simulink model "SimscapeFoundation_singleDiodeModel_solarCell"  (R2017b)
settings: Solver=FixedStepDiscrete  StartTime=0.0  StopTime=3.5  FixedStep=0.0001  MaxStep=1e-4  RelTol=1e-3
StopFcn:
  | run('plot_IV_curve')
undefined symbols (not defined in the file): physconst
libraries: fl_lib x5, nesl_utility x5, simulink x2
settings Model: Creator=Adrian  LastModifiedBy=Adrian

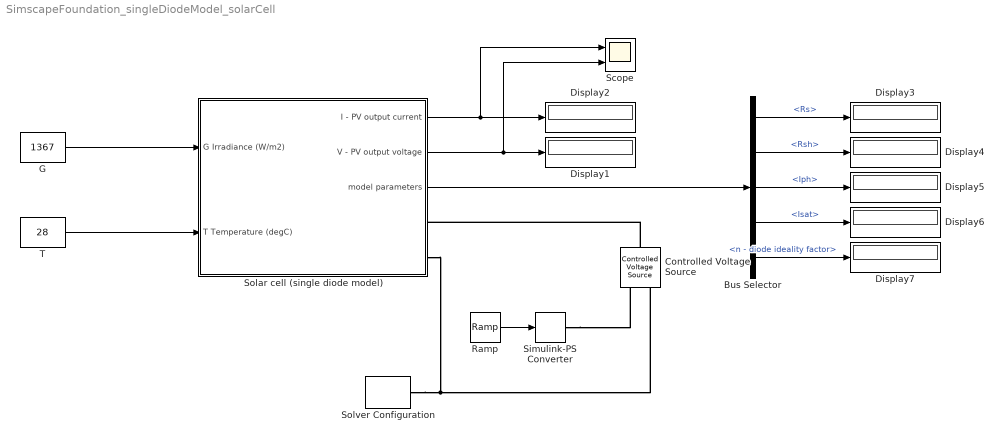
== system SimscapeFoundation_singleDiodeModel_solarCell ==
  Bus Selector : BusSelector  OutputSignals=Rs,Rsh,Iph,Isat,n - diode ideality factor
  Controlled Voltage Source : fl_lib/Electrical/Electrical Sources/Controlled Voltage Source
  Display{1..7} (7 alike) : Display
  G : Constant  Value=1367
  Ramp : simulink/Sources/Ramp  slope=1  start=0  X0=0
  Scope : Scope  NumInputPorts=2
  Simulink-PS Converter : nesl_utility/Simulink-PS Converter  PhysicalDomain=network_engine_domain  SubClassName=ps_input  LeftPortType=input  RightPortType=output  PseudoPeriodic=off  Frequencies=[]  NoiseDistribution=none  NoiseParameters=[]  Unit=1  AffineConversion=off  FilteringAndDerivatives=provide  SimscapeFilterOrder=1  InputFilterTimeConstant=0.001  UdotUserProvided=0
  Solar cell (single diode model) : Subsystem  mask(Solar cell model){T_ref=28, G_ref=1367, Voc_ref=2512, Isc_ref=501.3, Vmpp_ref=2244, Impp_ref=485.1, DVoc=-6.7, DVmpp=-7.2, DIsc=0.38, DImpp=0.28}
      mask prompts: T_ref "Temperature (degC), T_ref ="; G_ref "Irradiation (W/m2), G_ref ="; Voc_ref "Open circuit voltage (mV), Voc ="; Isc_ref "Short circuit current (mA), Isc ="; Vmpp_ref "Voltage @ mpp (mV), Vmpp ="; Impp_ref "Current @ mpp (mA), Impp ="; DVoc "Delta Voc / Delta T (mV/degC), DVoc ="; DVmpp "Delta Vmpp / Delta T (mV/degC), DVmpp ="; DIsc "Delta Isc / Delta T (mA/degC), DIsc ="; DImpp "Delta Impp / Delta T (mA/degC), DImpp ="
      mask help:
      | - "single diode + inner losses" solar cell model
      | - setup: current source, parallel diode, shunt and series resistor
      | - calculating the solar cell model's 5 parameters (Iph, Isat, n, Rsh, Rs, where n is already given) on every time step
      | - using those 5 parameters to control a parametrized current source
      | - input: irradiance, temperature
      | - model parameters get determined by using Voc, Isc, V and I @ mpp and the corresponding temperature dependencies of the given (modeled) solar cell
      mask TypeOptions T_ref: calculate 5 parameters of single diode solar cell model/T_ref
      mask TypeOptions G_ref: calculate 5 parameters of single diode solar cell model/G_ref
      mask TypeOptions Voc_ref: calculate 5 parameters of single diode solar cell model/Voc_ref
      mask TypeOptions Isc_ref: calculate 5 parameters of single diode solar cell model/Isc_ref
      mask TypeOptions Vmpp_ref: calculate 5 parameters of single diode solar cell model/Vmpp_ref
      mask TypeOptions Impp_ref: calculate 5 parameters of single diode solar cell model/Impp_ref
      mask TypeOptions DVoc: calculate 5 parameters of single diode solar cell model/DVoc
      mask TypeOptions DVmpp: calculate 5 parameters of single diode solar cell model/DVmpp
      mask TypeOptions DIsc: calculate 5 parameters of single diode solar cell model/DIsc
      mask TypeOptions DImpp: calculate 5 parameters of single diode solar cell model/DImpp
      mask DialogControl ParameterGroupVar Prompt: Conditions of reference measurement
      mask DialogControl Container3 Prompt: Characteristics (reference measurement @ T_ref, G_ref)
      mask DialogControl Container4 Prompt: Temperature dependencies
  Solver Configuration : nesl_utility/Solver Configuration  PhysicalDomain=network_engine_domain  SubClassName=solver  LeftPortType=input  RightPortType=generic  Accelerate=off  Tones=[]  Harmonics=[]  SimulateNoise=off  Profile=off  UseLocalSampling=off  EnableSwitchedLinearOptims=on  FrequencyDomain=off  UseCCode=off  RelTol=0.001  AbsTol=1e-06  MinStep=1e-09  ToWorkspace=off  RevertToSquareIcSolve=off  NumHomotopyIterations=100  PhasorMode=off  PhasorModeNumHarmonics=1  DoDC=off  ResidualTolerance=1e-09  UseLocalSolver=on  LocalSolverChoice=NE_BACKWARD_EULER_ADVANCER  LocalSolverSampleTime=0.001  DoFixedCost=on  MaxNonlinIter=3  MaxModeIter=2  LinearAlgebra=Sparse  DelaysMemoryBudget=1024  AutomaticFiltering=on  FilteringTimeConstant=0.001
  T : Constant  Value=28
  wires:
  G/1 -> Solar cell (single diode model)/1(G Irradiance (W/m2))
  T/1 -> Solar cell (single diode model)/2(T Temperature (degC))
  Solar cell (single diode model)/2(V - PV output voltage) -> Scope/2, Display1/1
  Solar cell (single diode model)/1(I - PV output current) -> Scope/1, Display2/1
  Ramp/1 -> Simulink-PS Converter/1
  Solar cell (single diode model)/3(model parameters) -> Bus Selector/1
  Bus Selector/1 -> Display3/1  "<Rs>"
  Bus Selector/2 -> Display4/1  "<Rsh>"
  Bus Selector/3 -> Display5/1  "<Iph>"
  Bus Selector/4 -> Display6/1  "<Isat>"
  Bus Selector/5 -> Display7/1  "<n - diode ideality factor>"
  connections:
  Controlled Voltage Source/LConn1 -- Solar cell (single diode model)/RConn1
  Solar cell (single diode model)/RConn2 -- Solver Configuration/RConn1 -- Controlled Voltage Source/RConn2
  Simulink-PS Converter/RConn1 -- Controlled Voltage Source/RConn1

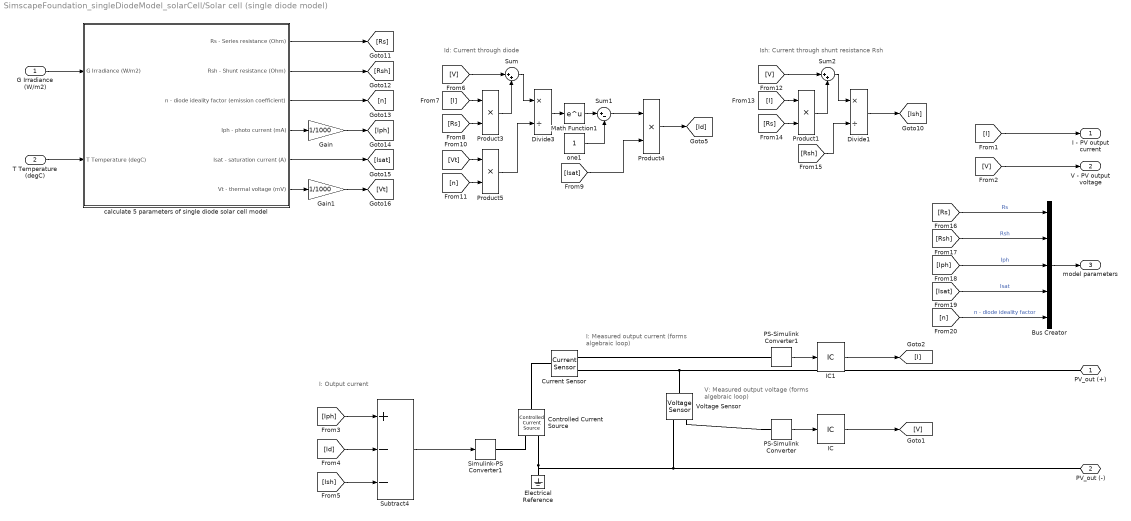
== system SimscapeFoundation_singleDiodeModel_solarCell/Solar cell (single diode model) ==
  note: Id: Current through diode
  note: Ish: Current through shunt resistance Rsh
  note: I: Output current
  note: I: Measured output current
      | (forms algebraic loop)
  note: V: Measured output voltage
      | (forms algebraic loop)
  G Irradiance (W/m2) : Inport
  T Temperature (degC) : Inport  Port=2
  Bus Creator : BusCreator  Inputs=5
  Controlled Current Source : fl_lib/Electrical/Electrical Sources/Controlled Current Source
  Current Sensor : fl_lib/Electrical/Electrical Sensors/Current Sensor
  Divide1 : Product  Inputs=*/
  Divide3 : Product  Inputs=*/
  Electrical Reference : fl_lib/Electrical/Electrical Elements/Electrical Reference
  Gain : Gain  Gain=1/1000
  Gain1 : Gain  Gain=1/1000
  IC : InitialCondition  Value=2.5
  IC1 : InitialCondition  Value=0.02
  Math Function1 : Math  SaturateOnIntegerOverflow=on
  PS-Simulink Converter : nesl_utility/PS-Simulink Converter  PhysicalDomain=network_engine_domain  SubClassName=ps_output  LeftPortType=input  RightPortType=output  PseudoPeriodic=off  Frequencies=[]  Unit=1  AffineConversion=off
  PS-Simulink Converter1 : nesl_utility/PS-Simulink Converter  PhysicalDomain=network_engine_domain  SubClassName=ps_output  LeftPortType=input  RightPortType=output  PseudoPeriodic=off  Frequencies=[]  Unit=1  AffineConversion=off
  Product{1,3..5} (4 alike) : Product
  Simulink-PS Converter1 : nesl_utility/Simulink-PS Converter  PhysicalDomain=network_engine_domain  SubClassName=ps_input  LeftPortType=input  RightPortType=output  PseudoPeriodic=off  Frequencies=[]  NoiseDistribution=none  NoiseParameters=[]  Unit=1  AffineConversion=off  FilteringAndDerivatives=provide  SimscapeFilterOrder=1  InputFilterTimeConstant=0.001  UdotUserProvided=0
  Subtract4 : Sum  Inputs=+--
  Sum : Sum  Inputs=|++
  Sum1 : Sum  Inputs=|+-
  Sum2 : Sum  Inputs=|++
  Voltage Sensor : fl_lib/Electrical/Electrical Sensors/Voltage Sensor
  calculate 5 parameters of single diode solar cell model : Subsystem  mask(Parameter identifier of "single diode" solar cell model){n=1.5, T_ref=T_ref, G_ref=G_ref, Voc_ref=Voc_ref, Isc_ref=Isc_ref, Vmpp_ref=Vmpp_ref, Impp_ref=Impp_ref, DVoc=DVoc, DVmpp=DVmpp, DIsc=DIsc, DImpp=DImpp}
      mask prompts: n "Diode ideality factor (emission coefficient)"; T_ref "Temperature (degC), T_ref ="; G_ref "Irradiation (W/m2), G_ref ="; Voc_ref "Open circuit voltage (mV), Voc ="; Isc_ref "Short circuit current (mA), Isc ="; Vmpp_ref "Voltage @ mpp (mV), Vmpp ="; Impp_ref "Current @ mpp (mA), Impp ="; DVoc "Delta Voc / Delta T (mV/degC), DVoc ="; DVmpp "Delta Vmpp / Delta T (mV/degC), DVmpp ="; DIsc "Delta Isc / Delta T (mA/degC), DIsc ="; DImpp "Delta Impp / Delta T (mA/degC), DImpp ="
      mask help:
      | - solar cell model, type: single diode + innert losses
      | - using a current source, parallel diode, shunt and series resistor
      | - output: 5 parameters (Iph, Isat, n, Rsh, Rs)
      | - input: irradiance, temperature
      | - model parameters get determined by using Voc, Isc, V and I @ mpp and the corresponding temperature dependencies
      mask DialogControl Container5 Prompt: Tunable model parameters
      mask DialogControl ParameterGroupVar Prompt: Conditions of reference measurement
      mask DialogControl Container8 Prompt: Characteristics (reference measurement @ T_ref, G_ref)
      mask DialogControl Container9 Prompt: Temperature dependencies
  one1 : Constant
  PV_out (+) : PMIOPort  Port=1  Side=Right
  PV_out (-) : PMIOPort  Port=2  Side=Right
  I - PV output current : Outport
  V - PV output voltage : Outport  Port=2
  model parameters : Outport  Port=3
  wires:
  Gain/1 -> [Iph]
  [I] -> Product1/1
  Product1/1 -> Sum2/2
  [V] -> Sum2/1
  [Id] -> Subtract4/2
  Divide3/1 -> Math Function1/1
  one1/1 -> Sum1/2
  Sum/1 -> Divide3/1
  [V] -> Sum/1
  [Ish] -> Subtract4/3
  Sum1/1 -> Product4/1
  Subtract4/1 -> Simulink-PS Converter1/1
  [Rs] -> Product1/2
  Product3/1 -> Sum/2
  PS-Simulink Converter/1 -> IC/1
  PS-Simulink Converter1/1 -> IC1/1
  Math Function1/1 -> Sum1/1
  [Isat] -> Product4/2
  [Rsh] -> Divide1/2
  Product4/1 -> [Id]
  [Vt] -> Product5/1
  [n] -> Product5/2
  [Iph] -> Subtract4/1
  [I] -> Product3/1
  Product5/1 -> Divide3/2
  IC/1 -> [V]
  IC1/1 -> [I]
  calculate 5 parameters of single diode solar cell model/6(Vt - thermal voltage (mV)) -> Gain1/1
  calculate 5 parameters of single diode solar cell model/4(Iph - photo current (mA)) -> Gain/1
  calculate 5 parameters of single diode solar cell model/1(Rs - Series resistance (Ohm)) -> [Rs]
  calculate 5 parameters of single diode solar cell model/5(Isat - saturation current (A)) -> [Isat]
  Sum2/1 -> Divide1/1
  Divide1/1 -> [Ish]
  calculate 5 parameters of single diode solar cell model/2(Rsh - Shunt resistance (Ohm)) -> [Rsh]
  T Temperature (degC)/1 -> calculate 5 parameters of single diode solar cell model/2(T Temperature (degC))
  Gain1/1 -> [Vt]
  [Rs] -> Product3/2
  G Irradiance (W/m2)/1 -> calculate 5 parameters of single diode solar cell model/1(G Irradiance (W/m2))
  calculate 5 parameters of single diode solar cell model/3(n - diode ideality factor (emission coefficient)) -> [n]
  [I] -> I - PV output current/1
  [V] -> V - PV output voltage/1
  [Rs] -> Bus Creator/1  "Rs"
  [Rsh] -> Bus Creator/2  "Rsh"
  [Iph] -> Bus Creator/3  "Iph"
  [Isat] -> Bus Creator/4  "Isat"
  Bus Creator/1 -> model parameters/1
  [n] -> Bus Creator/5  "n - diode ideality factor"
  connections:
  Controlled Current Source/LConn1 -- Current Sensor/LConn1
  Simulink-PS Converter1/RConn1 -- Controlled Current Source/RConn1
  Voltage Sensor/RConn2 -- PV_out (-)/RConn1 -- Electrical Reference/LConn1 -- Controlled Current Source/RConn2
  PS-Simulink Converter/LConn1 -- Voltage Sensor/RConn1
  Current Sensor/RConn2 -- Voltage Sensor/LConn1 -- PV_out (+)/RConn1
  Current Sensor/RConn1 -- PS-Simulink Converter1/LConn1

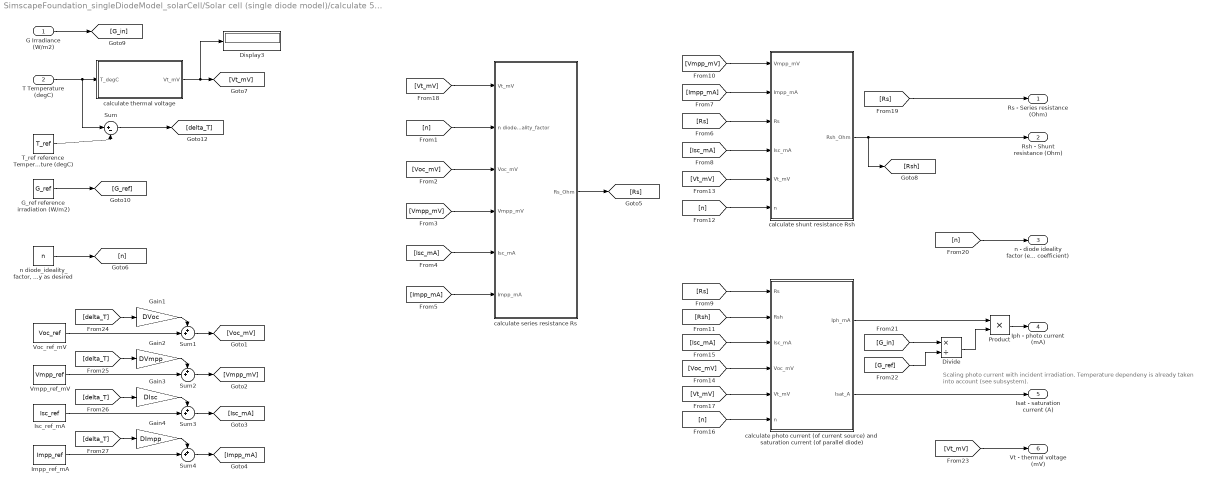
== system SimscapeFoundation_singleDiodeModel_solarCell/Solar cell (single diode model)/calculate 5 parameters of single diode solar cell model ==
  note: Scaling photo current with incident irradiation.
      | Temperature dependeny is already taken into account (see subsystem).
  G Irradiance (W/m2) : Inport
  T Temperature (degC) : Inport  Port=2
  Display3 : Display
  Divide : Product  Inputs=*/
  G_ref reference irradiation (W/m2) : Constant  Value=G_ref
  Gain1 : Gain  Gain=DVoc
  Gain2 : Gain  Gain=DVmpp
  Gain3 : Gain  Gain=DIsc
  Gain4 : Gain  Gain=DImpp
  Impp_ref_mA : Constant  Value=Impp_ref
  Isc_ref_mA : Constant  Value=Isc_ref
  Product : Product
  Sum : Sum  Inputs=|+-
  Sum{1..4} (4 alike) : Sum  Inputs=++|
  T_ref reference Temperature (degC) : Constant  Value=T_ref
  Vmpp_ref_mV : Constant  Value=Vmpp_ref
  Voc_ref_mV : Constant  Value=Voc_ref
  calculate photo current (of current source) and saturation current (of parallel diode) : Subsystem
  calculate series resistance Rs : Subsystem
  calculate shunt resistance Rsh : Subsystem
  calculate thermal voltage : Subsystem
  "n diode_ideality_factor, normally 1...2 specify as desired " : Constant  Value=n
  Rs - Series resistance (Ohm) : Outport
  Rsh - Shunt resistance (Ohm) : Outport  Port=2
  n - diode ideality factor (emission coefficient) : Outport  Port=3
  Iph - photo current (mA) : Outport  Port=4
  Isat - saturation current (A) : Outport  Port=5
  Vt - thermal voltage (mV) : Outport  Port=6
  wires:
  [Vt_mV] -> calculate series resistance Rs/1(Vt_mV)
  [Impp_mA] -> calculate series resistance Rs/6(Impp_mA)
  [Vmpp_mV] -> calculate series resistance Rs/4(Vmpp_mV)
  [Isc_mA] -> calculate series resistance Rs/5(Isc_mA)
  [Voc_mV] -> calculate series resistance Rs/3(Voc_mV)
  calculate thermal voltage/1(Vt_mV) -> Display3/1, [Vt_mV]
  [n] -> calculate series resistance Rs/2(n diode_ideality_factor)
  calculate series resistance Rs/1(Rs_Ohm) -> [Rs]
  "n diode_ideality_factor, normally 1...2 specify as desired "/1 -> [n]
  [n] -> calculate shunt resistance Rsh/6(n)
  [Rs] -> calculate photo current (of current source) and saturation current (of parallel diode)/1(Rs)
  calculate photo current (of current source) and saturation current (of parallel diode)/2(Isat_A) -> Isat - saturation current (A)/1
  [Voc_mV] -> calculate photo current (of current source) and saturation current (of parallel diode)/4(Voc_mV)
  [Impp_mA] -> calculate shunt resistance Rsh/2(Impp_mA)
  [Vt_mV] -> calculate shunt resistance Rsh/5(Vt_mV)
  [Vt_mV] -> calculate photo current (of current source) and saturation current (of parallel diode)/5(Vt_mV)
  [Rs] -> calculate shunt resistance Rsh/3(Rs)
  [Isc_mA] -> calculate shunt resistance Rsh/4(Isc_mA)
  [Vmpp_mV] -> calculate shunt resistance Rsh/1(Vmpp_mV)
  [Isc_mA] -> calculate photo current (of current source) and saturation current (of parallel diode)/3(Isc_mA)
  [n] -> calculate photo current (of current source) and saturation current (of parallel diode)/6(n)
  [Rsh] -> calculate photo current (of current source) and saturation current (of parallel diode)/2(Rsh)
  calculate shunt resistance Rsh/1(Rsh_Ohm) -> Rsh - Shunt resistance (Ohm)/1, [Rsh]
  calculate photo current (of current source) and saturation current (of parallel diode)/1(Iph_mA) -> Product/1
  T Temperature (degC)/1 -> Sum/1, calculate thermal voltage/1(T_degC)
  [Rs] -> Rs - Series resistance (Ohm)/1
  G Irradiance (W/m2)/1 -> [G_in]
  [G_in] -> Divide/1
  [n] -> n - diode ideality factor (emission coefficient)/1
  Product/1 -> Iph - photo current (mA)/1
  G_ref reference irradiation (W/m2)/1 -> [G_ref]
  Divide/1 -> Product/2
  [G_ref] -> Divide/2
  [Vt_mV] -> Vt - thermal voltage (mV)/1
  T_ref reference Temperature (degC)/1 -> Sum/2
  Sum/1 -> [delta_T]
  [delta_T] -> Gain1/1
  Voc_ref_mV/1 -> Sum1/2
  Sum1/1 -> [Voc_mV]
  Gain1/1 -> Sum1/1
  Gain2/1 -> Sum2/1
  Sum2/1 -> [Vmpp_mV]
  Vmpp_ref_mV/1 -> Sum2/2
  [delta_T] -> Gain2/1
  [delta_T] -> Gain4/1
  Impp_ref_mA/1 -> Sum4/2
  Sum4/1 -> [Impp_mA]
  Gain4/1 -> Sum4/1
  Gain3/1 -> Sum3/1
  Sum3/1 -> [Isc_mA]
  Isc_ref_mA/1 -> Sum3/2
  [delta_T] -> Gain3/1

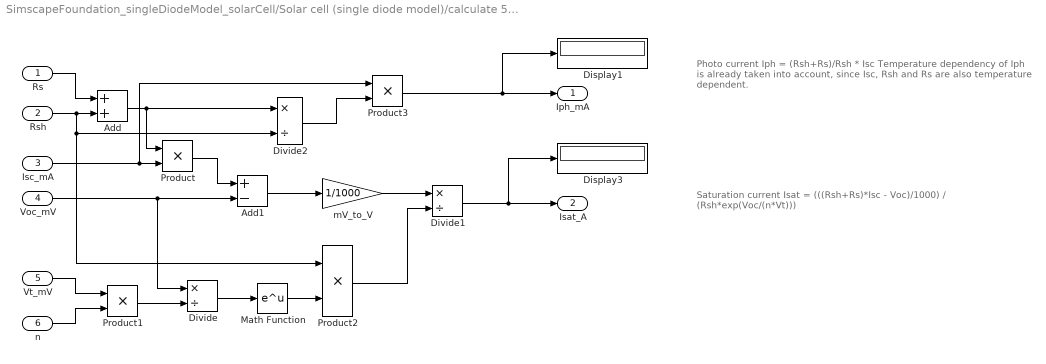
== system SimscapeFoundation_singleDiodeModel_solarCell/Solar cell (single diode model)/calculate 5 parameters of single diode solar cell model/calculate photo current (of current source) and saturation current (of parallel diode) ==
  note: Saturation current
      | Isat = (((Rsh+Rs)*Isc - Voc)/1000) / (Rsh*exp(Voc/(n*Vt)))
  note: Photo current
      | Iph = (Rsh+Rs)/Rsh * Isc
      |
      | Temperature dependency of Iph is already taken into account,
      | since Isc, Rsh and Rs are also temperature dependent.
  Rs : Inport
  Rsh : Inport  Port=2
  Isc_mA : Inport  Port=3
  Voc_mV : Inport  Port=4
  Vt_mV : Inport  Port=5
  n : Inport  Port=6
  Add : Sum
  Add1 : Sum  Inputs=+-
  Display1 : Display
  Display3 : Display
  Divide : Product  Inputs=*/
  Divide1 : Product  Inputs=*/
  Divide2 : Product  Inputs=*/
  Math Function : Math  SaturateOnIntegerOverflow=on
  Product{,1..3} (4 alike) : Product
  mV_to_V : Gain  Gain=1/1000
  Iph_mA : Outport
  Isat_A : Outport  Port=2
  wires:
  Product2/1 -> Divide1/2
  Isc_mA/1 -> Product3/1, Product/2
  Divide/1 -> Math Function/1
  Voc_mV/1 -> Add1/2, Divide/1
  Product1/1 -> Divide/2
  Vt_mV/1 -> Product1/1
  Rs/1 -> Add/1
  Add1/1 -> mV_to_V/1
  n/1 -> Product1/2
  Divide1/1 -> Display3/1, Isat_A/1
  Product/1 -> Add1/1
  Rsh/1 -> Divide2/2, Product2/1, Add/2
  mV_to_V/1 -> Divide1/1
  Add/1 -> Product/1, Divide2/1
  Math Function/1 -> Product2/2
  Divide2/1 -> Product3/2
  Product3/1 -> Display1/1, Iph_mA/1

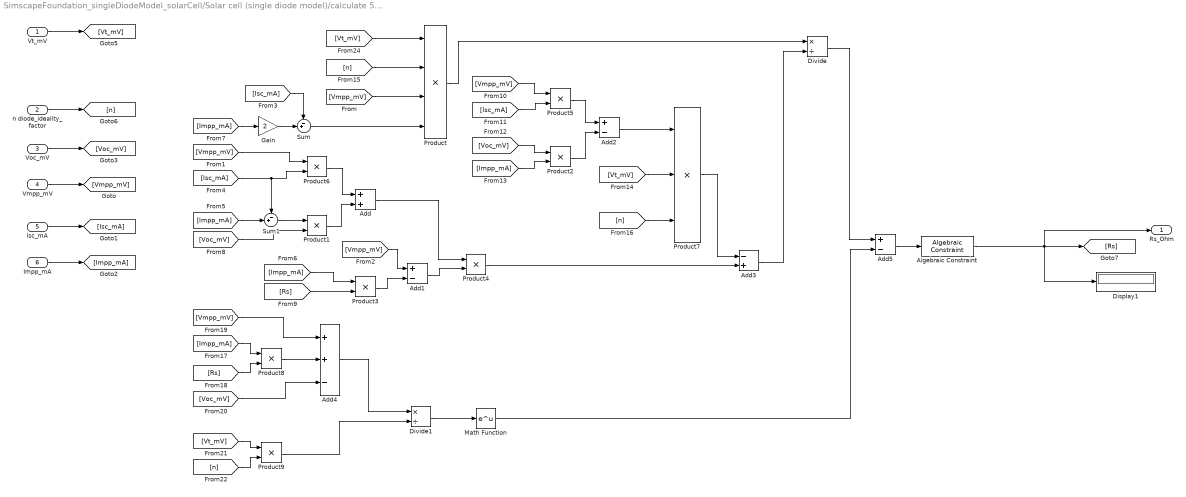
== system SimscapeFoundation_singleDiodeModel_solarCell/Solar cell (single diode model)/calculate 5 parameters of single diode solar cell model/calculate series resistance Rs ==
  Vt_mV : Inport
  n diode_ideality_factor : Inport  Port=2
  Voc_mV : Inport  Port=3
  Vmpp_mV : Inport  Port=4
  Isc_mA : Inport  Port=5
  Impp_mA : Inport  Port=6
  Add : Sum
  Add1 : Sum  Inputs=+-
  Add2 : Sum  Inputs=+-
  Add3 : Sum  Inputs=-+
  Add4 : Sum  Inputs=++-
  Add5 : Sum  Inputs=+-
  Algebraic Constraint : simulink/Math Operations/Algebraic Constraint  z0=0
      settings: SourceProductName=Simulink  SourceProductBaseCode=SL
  Display1 : Display
  Divide : Product  Inputs=*/
  Divide1 : Product  Inputs=*/
  Gain : Gain  Gain=2
  Math Function : Math  SaturateOnIntegerOverflow=on
  Product : Product  Inputs=4
  Product{1..6,8..9} (8 alike) : Product
  Product7 : Product  Inputs=3
  Sum : Sum  Inputs=-+|
  Sum1 : Sum  Inputs=-+|
  Rs_Ohm : Outport
  wires:
  [Vmpp_mV] -> Add1/1
  Vmpp_mV/1 -> [Vmpp_mV]
  [Voc_mV] -> Add4/3
  Product7/1 -> Add3/1
  [Voc_mV] -> Product1/2
  [Vt_mV] -> Product/1
  [Voc_mV] -> Product2/1
  [Vmpp_mV] -> Add4/1
  Gain/1 -> Sum/2
  Product2/1 -> Add2/2
  [Vmpp_mV] -> Product/3
  Divide/1 -> Add5/1
  Product9/1 -> Divide1/2
  [n] -> Product/2
  [Vt_mV] -> Product7/2
  [Vmpp_mV] -> Product5/1
  [Impp_mA] -> Product8/1
  [Impp_mA] -> Sum1/2
  [Vmpp_mV] -> Product6/1
  Product5/1 -> Add2/1
  [Isc_mA] -> Sum/1
  [Impp_mA] -> Gain/1
  [Rs] -> Product3/2
  [n] -> Product7/3
  [Impp_mA] -> Product3/1
  Add/1 -> Product4/1
  Add2/1 -> Product7/1
  Divide1/1 -> Math Function/1
  n diode_ideality_factor/1 -> [n]
  Product1/1 -> Add/2
  Sum/1 -> Product/4
  [Vt_mV] -> Product9/1
  Add5/1 -> Algebraic Constraint/1
  Add3/1 -> Divide/2
  [Isc_mA] -> Product5/2
  Product6/1 -> Add/1
  Vt_mV/1 -> [Vt_mV]
  Impp_mA/1 -> [Impp_mA]
  Isc_mA/1 -> [Isc_mA]
  Product3/1 -> Add1/2
  Sum1/1 -> Product1/1
  Voc_mV/1 -> [Voc_mV]
  Product8/1 -> Add4/2
  Add1/1 -> Product4/2
  Product/1 -> Divide/1
  [Rs] -> Product8/2
  [n] -> Product9/2
  [Impp_mA] -> Product2/2
  Add4/1 -> Divide1/1
  [Isc_mA] -> Sum1/1, Product6/2
  Algebraic Constraint/1 -> Rs_Ohm/1, [Rs], Display1/1
  Math Function/1 -> Add5/2
  Product4/1 -> Add3/2

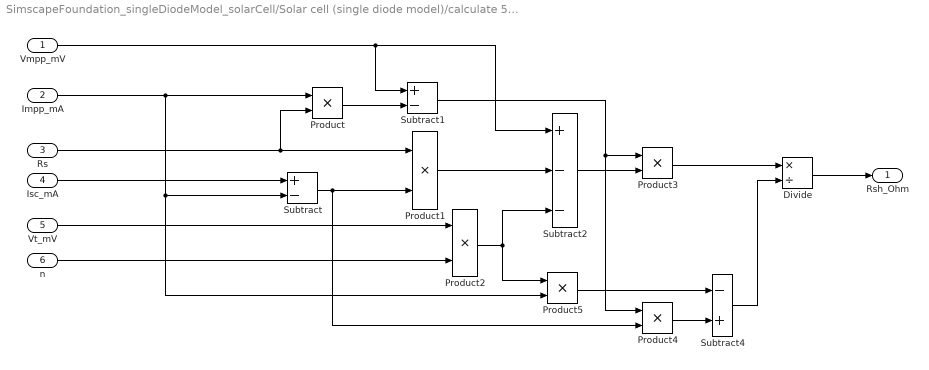
== system SimscapeFoundation_singleDiodeModel_solarCell/Solar cell (single diode model)/calculate 5 parameters of single diode solar cell model/calculate shunt resistance Rsh ==
  Vmpp_mV : Inport
  Impp_mA : Inport  Port=2
  Rs : Inport  Port=3
  Isc_mA : Inport  Port=4
  Vt_mV : Inport  Port=5
  n : Inport  Port=6
  Divide : Product  Inputs=*/
  Product{,1..5} (6 alike) : Product
  Subtract : Sum  Inputs=+-
  Subtract1 : Sum  Inputs=+-
  Subtract2 : Sum  Inputs=+--
  Subtract4 : Sum  Inputs=-+
  Rsh_Ohm : Outport
  wires:
  Subtract4/1 -> Divide/2
  Product3/1 -> Divide/1
  Product5/1 -> Subtract4/1
  Rs/1 -> Product/2, Product1/1
  Isc_mA/1 -> Subtract/1
  Product1/1 -> Subtract2/2
  Vmpp_mV/1 -> Subtract1/1, Subtract2/1
  n/1 -> Product2/2
  Vt_mV/1 -> Product2/1
  Subtract1/1 -> Product4/1, Product3/1
  Divide/1 -> Rsh_Ohm/1
  Product2/1 -> Subtract2/3, Product5/1
  Subtract/1 -> Product1/2, Product4/2
  Product/1 -> Subtract1/2
  Subtract2/1 -> Product3/2
  Product4/1 -> Subtract4/2
  Impp_mA/1 -> Subtract/2, Product5/2, Product/1

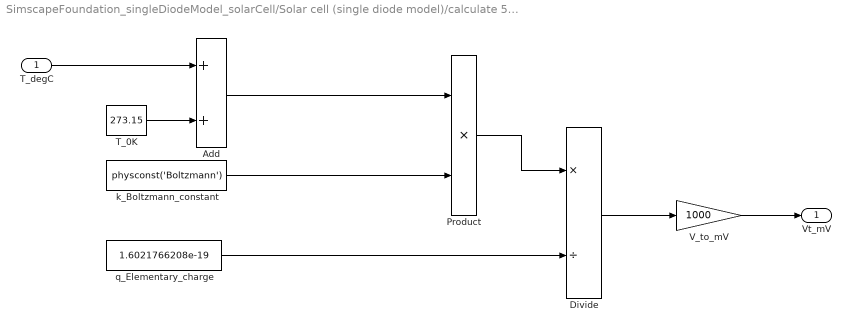
== system SimscapeFoundation_singleDiodeModel_solarCell/Solar cell (single diode model)/calculate 5 parameters of single diode solar cell model/calculate thermal voltage ==
  T_degC : Inport
  Add : Sum
  Divide : Product  Inputs=*/
  Product : Product
  T_0K : Constant  Value=273.15
  V_to_mV : Gain  Gain=1000
  k_Boltzmann_constant : Constant  Value=physconst('Boltzmann')
  q_Elementary_charge : Constant  Value=1.6021766208e-19
  Vt_mV : Outport
  wires:
  Product/1 -> Divide/1
  Divide/1 -> V_to_mV/1
  k_Boltzmann_constant/1 -> Product/2
  V_to_mV/1 -> Vt_mV/1
  q_Elementary_charge/1 -> Divide/2
  Add/1 -> Product/1
  T_degC/1 -> Add/1
  T_0K/1 -> Add/2
